simulink model "TC_RT2004_pois_CX_SNr"  (R2016b)
settings: Solver=ode4  StartTime=0.0  StopTime=simtime  FixedStep=stepsize  MaxStep=stepsize  RelTol=1e-2  EnableMultiTasking=on
values from neighbouring files (symbols this model uses):
  alphaSNrtoTH = 5    [TC_model_CX_SNr_cond_changed_parfor_opt.m]
  apr = 4    [TC_model_CX_SNr_cond_changed_parfor_opt.m]
  apt = 0.3    [TC_model_CX_SNr_cond_changed_parfor_opt.m]
  betaSNrtoTH = 0.18    [TC_model_CX_SNr_cond_changed_parfor_opt.m]
  ek = -90    [TC_model_CX_SNr_cond_changed_parfor_opt.m]
  eleak = -70    [TC_model_CX_SNr_cond_changed_parfor_opt.m]
  ena = 50    [TC_model_CX_SNr_cond_changed_parfor_opt.m]
  gkbar = 5    [TC_model_CX_SNr_cond_changed_parfor_opt.m]
  glbar = 0.05    [TC_model_CX_SNr_cond_changed_parfor_opt.m]
  gnabar = 3    [TC_model_CX_SNr_cond_changed_parfor_opt.m]
  gsynSNrtoTH = g_snr    [TC_model_CX_SNr_cond_changed_parfor_opt.m]
  gtbar = 5    [TC_model_CX_SNr_cond_changed_parfor_opt.m]
  ht0 = 0    [TC_model_CX_SNr_cond_changed_parfor_opt.m]
  htt0 = 0    [TC_model_CX_SNr_cond_changed_parfor_opt.m]
  qht = 5.5    [TC_model_CX_SNr_cond_changed_parfor_opt.m]
  s0SNrtoTH = 0    [TC_model_CX_SNr_cond_changed_parfor_opt.m]
  tadj = 1    [TC_model_CX_SNr_cond_changed_parfor_opt.m]
  vsynSNrtoTH = -85    [TC_model_CX_SNr_cond_changed_parfor_opt.m]
  vt0 = 0    [TC_model_CX_SNr_cond_changed_parfor_opt.m]
undefined symbols (not defined in the file or in its folder): jit_spk_times
settings Model: Creator=mohaghegh  LastModifiedBy=Mohammad
settings SolverCC: ZeroCrossAlgorithm=Adaptive
settings DataIOCC: LimitDataPoints=on  SaveFormat=Array
settings OptimizationCC: LifeSpan=inf
settings DebuggingCC: SolverPrmCheckMsg=warning  SFUnexpectedBacktrackingDiag=warning  SFNoUnconditionalDefaultTransitionDiag=warning  SFExecutionAtInitializationDiag=none
settings HardwareCC: ProdBitPerPointer=32  ProdBitPerSizeT=32  ProdBitPerPtrDiffT=32  ProdLargestAtomicFloat=None  ProdIntDivRoundTo=Undefined  ProdEndianess=Unspecified  ProdWordSize=32  ProdHWDeviceType=32-bit Generic
settings ModelReferenceCC: PropagateSignalLabelsOutOfModel=off
settings GRTTargetCC: TargetLangStandard=C89/C90 (ANSI)  GeneratePreprocessorConditionals=Disable all
settings ConfigComp: CovMetricSettings=dw  CovHtmlReporting=on  CovSaveCumulativeToWorkspaceVar=on  CovSaveSingleToWorkspaceVar=on  CovExternalEMLEnable=off  CovSFcnEnable=off

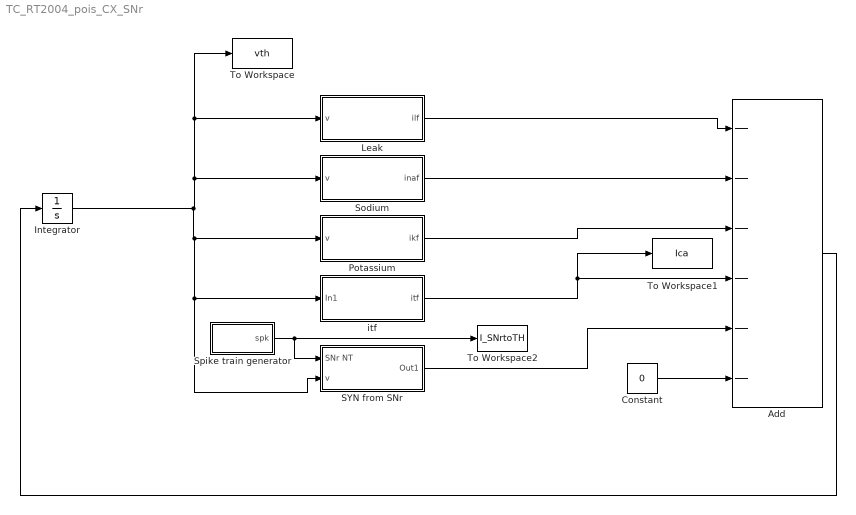
== system TC_RT2004_pois_CX_SNr ==
  Add : Sum  Inputs=------
  Constant : Constant  Value=0
  Integrator : Integrator  InitialCondition=vt0
  Leak : Subsystem
  Potassium : Subsystem
  SYN from SNr : Subsystem
  Sodium : Subsystem
  Spike train generator : Subsystem
  To Workspace : ToWorkspace  VariableName=vth  SaveFormat=Structure With Time  SampleTime=-1
  To Workspace1 : ToWorkspace  VariableName=Ica  SaveFormat=Structure With Time  SampleTime=-1
  To Workspace2 : ToWorkspace  VariableName=I_SNrtoTH  SaveFormat=Structure With Time  SampleTime=-1
  itf : Subsystem
  wires:
  Add/1 -> Integrator/1
  Leak/1(ilf) -> Add/1
  Sodium/1(inaf) -> Add/2
  Potassium/1(ikf) -> Add/3
  Integrator/1 -> SYN from SNr/2(v), itf/1(In1), Potassium/1(v), Sodium/1(v), To Workspace/1, Leak/1(v)
  SYN from SNr/1(Out1) -> Add/5
  Spike train generator/1(spk) -> To Workspace2/1, SYN from SNr/1(SNr NT)
  itf/1(itf) -> To Workspace1/1, Add/4
  Constant/1 -> Add/6

== system TC_RT2004_pois_CX_SNr/Leak ==
  v : Inport
  Constant : Constant  Value=eleak
  Gain : Gain  Gain=glbar
  Subtract : Sum  Inputs=+-
  ilf : Outport
  wires:
  v/1 -> Subtract/1
  Constant/1 -> Subtract/2
  Subtract/1 -> Gain/1
  Gain/1 -> ilf/1

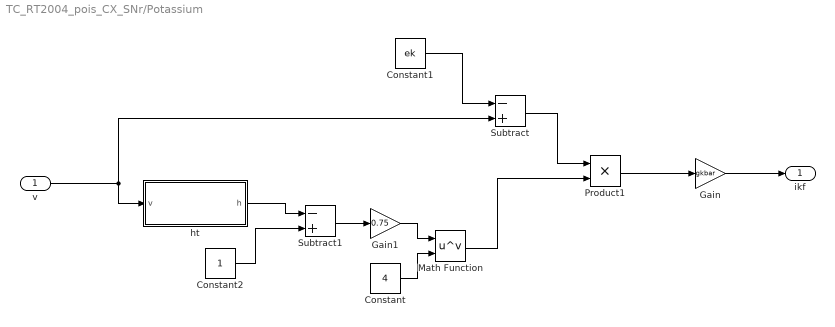
== system TC_RT2004_pois_CX_SNr/Potassium ==
  v : Inport
  Constant : Constant  Value=4
  Constant1 : Constant  Value=ek
  Constant2 : Constant
  Gain : Gain  Gain=gkbar
  Gain1 : Gain  Gain=0.75
  Math Function : Math  Operator=pow  SaturateOnIntegerOverflow=on
  Product1 : Product
  Subtract : Sum  Inputs=-+
  Subtract1 : Sum  Inputs=-+
  ht : Subsystem
  ikf : Outport
  wires:
  Gain/1 -> ikf/1
  Product1/1 -> Gain/1
  Subtract/1 -> Product1/1
  Constant1/1 -> Subtract/1
  Constant/1 -> Math Function/2
  v/1 -> ht/1(v), Subtract/2
  Math Function/1 -> Product1/2
  ht/1(h) -> Subtract1/1
  Constant2/1 -> Subtract1/2
  Subtract1/1 -> Gain1/1
  Gain1/1 -> Math Function/1

== system TC_RT2004_pois_CX_SNr/SYN from SNr ==
  SNr NT : Inport
  v : Inport  Port=2
  Add1 : Sum  Inputs=-+
  Constant : Constant  Value=vsynSNrtoTH
  Gain : Gain  Gain=gsynSNrtoTH
  Product : Product
  SNr to TH : Subsystem
  Out1 : Outport
  wires:
  Constant/1 -> Add1/1
  v/1 -> Add1/2
  Add1/1 -> Product/1
  Product/1 -> Gain/1
  Gain/1 -> Out1/1
  SNr NT/1 -> SNr to TH/1(s SNr)
  SNr to TH/1(SNr to TH cond) -> Product/2

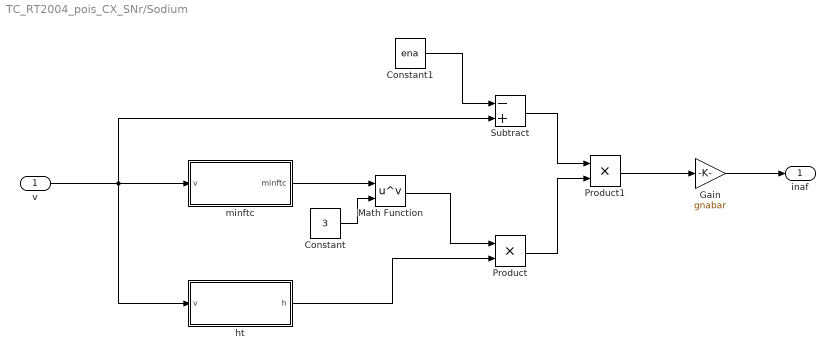
== system TC_RT2004_pois_CX_SNr/Sodium ==
  v : Inport
  Constant : Constant  Value=3
  Constant1 : Constant  Value=ena
  Gain : Gain  Gain=gnabar
  Math Function : Math  Operator=pow  SaturateOnIntegerOverflow=on
  Product : Product
  Product1 : Product
  Subtract : Sum  Inputs=-+
  ht : Subsystem
  minftc : Subsystem
  inaf : Outport
  wires:
  v/1 -> ht/1(v), minftc/1(v), Subtract/2
  minftc/1(minftc) -> Math Function/1
  Constant/1 -> Math Function/2
  Math Function/1 -> Product/1
  ht/1(h) -> Product/2
  Constant1/1 -> Subtract/1
  Subtract/1 -> Product1/1
  Product/1 -> Product1/2
  Product1/1 -> Gain/1
  Gain/1 -> inaf/1

== system TC_RT2004_pois_CX_SNr/Spike train generator ==
  Clock : Clock
  Constant : Constant  Value=jit_spk_times
  MATLAB Function : MATLAB Function  TreatAsAtomicUnit=on
  Memory : Memory
  spk : Outport
  wires:
  Clock/1 -> Memory/1, MATLAB Function/1(t1)
  Memory/1 -> MATLAB Function/2(t2)
  Constant/1 -> MATLAB Function/3(spks)
  MATLAB Function/1(y) -> spk/1

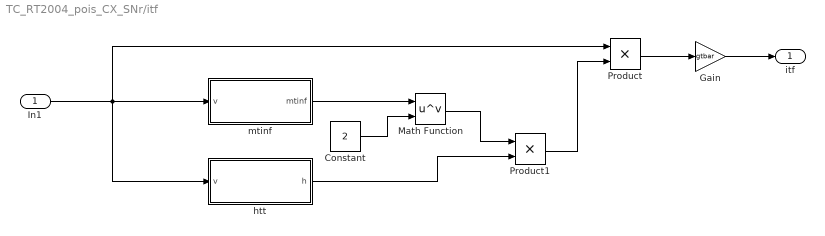
== system TC_RT2004_pois_CX_SNr/itf ==
  In1 : Inport
  Constant : Constant  Value=2
  Gain : Gain  Gain=gtbar
  Math Function : Math  Operator=pow  SaturateOnIntegerOverflow=on
  Product : Product
  Product1 : Product
  htt : Subsystem
  mtinf : Subsystem
  itf : Outport
  wires:
  In1/1 -> Product/1, mtinf/1(v), htt/1(v)
  mtinf/1(mtinf) -> Math Function/1
  Constant/1 -> Math Function/2
  Math Function/1 -> Product1/1
  htt/1(h) -> Product1/2
  Product1/1 -> Product/2
  Product/1 -> Gain/1
  Gain/1 -> itf/1

== system TC_RT2004_pois_CX_SNr/Potassium/ht ==
  v : Inport
  Divide : Product  Inputs=*/
  Gain : Gain  Gain=tadj
  Integrator : Integrator  InitialCondition=ht0
  Subtract : Sum  Inputs=-+
  hinftc : Subsystem
  tauhtc : Subsystem
  h : Outport
  wires:
  Gain/1 -> Integrator/1
  Divide/1 -> Gain/1
  tauhtc/1(tauhtc) -> Divide/2
  Subtract/1 -> Divide/1
  hinftc/1(hinftc) -> Subtract/2
  Integrator/1 -> h/1, Subtract/1
  v/1 -> tauhtc/1(v), hinftc/1(v)

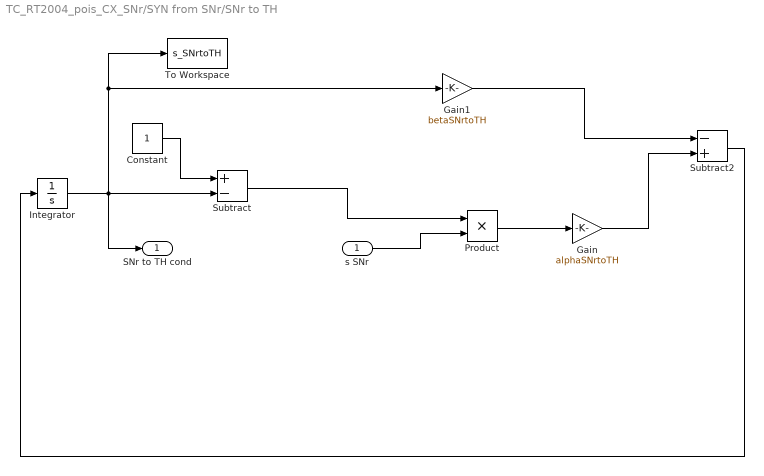
== system TC_RT2004_pois_CX_SNr/SYN from SNr/SNr to TH ==
  s SNr : Inport
  Constant : Constant
  Gain : Gain  Gain=alphaSNrtoTH
  Gain1 : Gain  Gain=betaSNrtoTH
  Integrator : Integrator  InitialCondition=s0SNrtoTH
  Product : Product
  Subtract : Sum  Inputs=+-
  Subtract2 : Sum  Inputs=-+
  To Workspace : ToWorkspace  VariableName=s_SNrtoTH  SaveFormat=Structure With Time  SampleTime=-1
  SNr to TH cond : Outport
  wires:
  Constant/1 -> Subtract/1
  Integrator/1 -> SNr to TH cond/1, To Workspace/1, Gain1/1, Subtract/2
  Subtract/1 -> Product/1
  Product/1 -> Gain/1
  Gain1/1 -> Subtract2/1
  Gain/1 -> Subtract2/2
  Subtract2/1 -> Integrator/1
  s SNr/1 -> Product/2

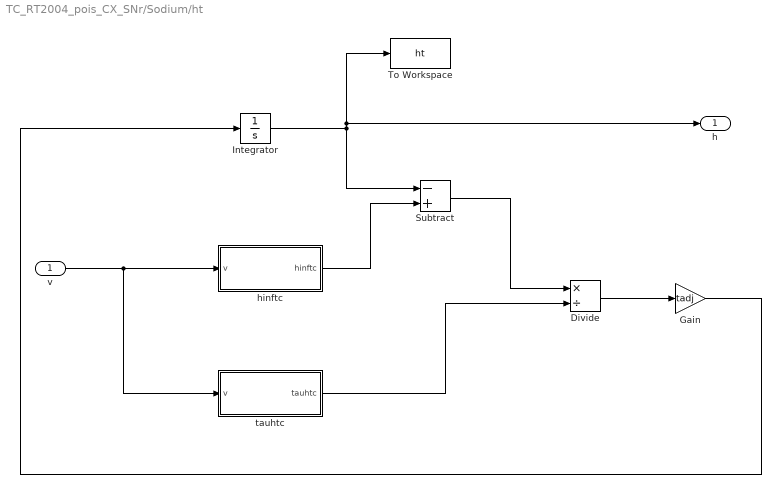
== system TC_RT2004_pois_CX_SNr/Sodium/ht ==
  v : Inport
  Divide : Product  Inputs=*/
  Gain : Gain  Gain=tadj
  Integrator : Integrator  InitialCondition=ht0
  Subtract : Sum  Inputs=-+
  To Workspace : ToWorkspace  VariableName=ht  SaveFormat=Structure With Time  SampleTime=-1
  hinftc : Subsystem
  tauhtc : Subsystem
  h : Outport
  wires:
  Gain/1 -> Integrator/1
  Divide/1 -> Gain/1
  tauhtc/1(tauhtc) -> Divide/2
  Subtract/1 -> Divide/1
  hinftc/1(hinftc) -> Subtract/2
  Integrator/1 -> To Workspace/1, h/1, Subtract/1
  v/1 -> tauhtc/1(v), hinftc/1(v)

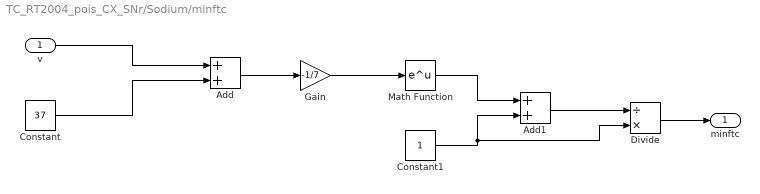
== system TC_RT2004_pois_CX_SNr/Sodium/minftc ==
  v : Inport
  Add : Sum
  Add1 : Sum
  Constant : Constant  Value=37
  Constant1 : Constant
  Divide : Product  Inputs=/*
  Gain : Gain  Gain=-1/7
  Math Function : Math  SaturateOnIntegerOverflow=on
  minftc : Outport
  wires:
  v/1 -> Add/1
  Constant/1 -> Add/2
  Add/1 -> Gain/1
  Gain/1 -> Math Function/1
  Math Function/1 -> Add1/1
  Add1/1 -> Divide/1
  Constant1/1 -> Divide/2, Add1/2
  Divide/1 -> minftc/1

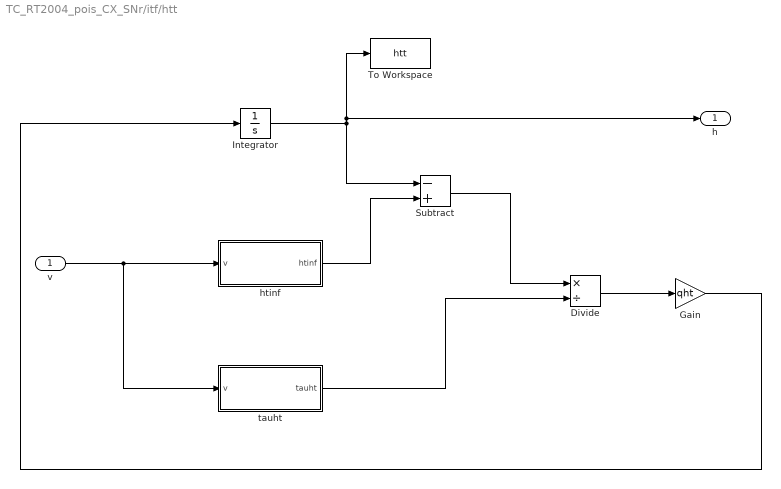
== system TC_RT2004_pois_CX_SNr/itf/htt ==
  v : Inport
  Divide : Product  Inputs=*/
  Gain : Gain  Gain=qht
  Integrator : Integrator  InitialCondition=htt0
  Subtract : Sum  Inputs=-+
  To Workspace : ToWorkspace  VariableName=htt  SaveFormat=Structure With Time  SampleTime=-1
  htinf : Subsystem
  tauht : Subsystem
  h : Outport
  wires:
  v/1 -> tauht/1(v), htinf/1(v)
  Integrator/1 -> To Workspace/1, h/1, Subtract/1
  htinf/1(htinf) -> Subtract/2
  Subtract/1 -> Divide/1
  tauht/1(tauht) -> Divide/2
  Divide/1 -> Gain/1
  Gain/1 -> Integrator/1

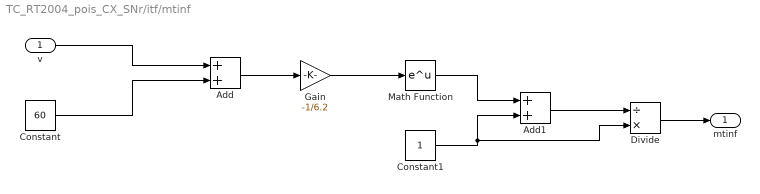
== system TC_RT2004_pois_CX_SNr/itf/mtinf ==
  v : Inport
  Add : Sum
  Add1 : Sum
  Constant : Constant  Value=60
  Constant1 : Constant
  Divide : Product  Inputs=/*
  Gain : Gain  Gain=-1/6.2
  Math Function : Math  SaturateOnIntegerOverflow=on
  mtinf : Outport
  wires:
  Divide/1 -> mtinf/1
  Constant1/1 -> Add1/2, Divide/2
  Add1/1 -> Divide/1
  Math Function/1 -> Add1/1
  Gain/1 -> Math Function/1
  Add/1 -> Gain/1
  Constant/1 -> Add/2
  v/1 -> Add/1

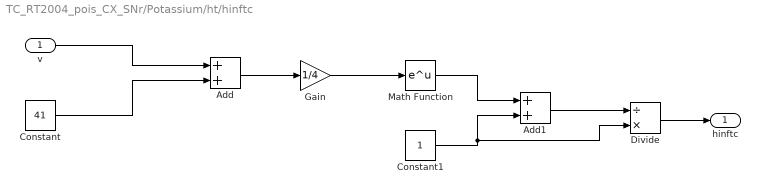
== system TC_RT2004_pois_CX_SNr/Potassium/ht/hinftc ==
  v : Inport
  Add : Sum
  Add1 : Sum
  Constant : Constant  Value=41
  Constant1 : Constant
  Divide : Product  Inputs=/*
  Gain : Gain  Gain=1/4
  Math Function : Math  SaturateOnIntegerOverflow=on
  hinftc : Outport
  wires:
  v/1 -> Add/1
  Constant/1 -> Add/2
  Add/1 -> Gain/1
  Gain/1 -> Math Function/1
  Math Function/1 -> Add1/1
  Add1/1 -> Divide/1
  Constant1/1 -> Divide/2, Add1/2
  Divide/1 -> hinftc/1

== system TC_RT2004_pois_CX_SNr/Potassium/ht/tauhtc ==
  v : Inport
  Add : Sum
  Constant : Constant
  Divide : Product  Inputs=*/
  ah : Subsystem
  bh : Subsystem
  tauhtc : Outport
  wires:
  v/1 -> bh/1(v), ah/1(v)
  ah/1(ah) -> Add/1
  bh/1(bh) -> Add/2
  Constant/1 -> Divide/1
  Add/1 -> Divide/2
  Divide/1 -> tauhtc/1

== system TC_RT2004_pois_CX_SNr/Sodium/ht/hinftc ==
  v : Inport
  Add : Sum
  Add1 : Sum
  Constant : Constant  Value=41
  Constant1 : Constant
  Divide : Product  Inputs=/*
  Gain : Gain  Gain=1/4
  Math Function : Math  SaturateOnIntegerOverflow=on
  hinftc : Outport
  wires:
  v/1 -> Add/1
  Constant/1 -> Add/2
  Add/1 -> Gain/1
  Gain/1 -> Math Function/1
  Math Function/1 -> Add1/1
  Add1/1 -> Divide/1
  Constant1/1 -> Divide/2, Add1/2
  Divide/1 -> hinftc/1

== system TC_RT2004_pois_CX_SNr/Sodium/ht/tauhtc ==
  v : Inport
  Add : Sum
  Constant : Constant
  Divide : Product  Inputs=*/
  ah : Subsystem
  bh : Subsystem
  tauhtc : Outport
  wires:
  v/1 -> bh/1(v), ah/1(v)
  ah/1(ah) -> Add/1
  bh/1(bh) -> Add/2
  Constant/1 -> Divide/1
  Add/1 -> Divide/2
  Divide/1 -> tauhtc/1

== system TC_RT2004_pois_CX_SNr/itf/htt/htinf ==
  v : Inport
  Add : Sum
  Add1 : Sum
  Constant : Constant  Value=84
  Constant1 : Constant
  Divide : Product  Inputs=/*
  Gain : Gain  Gain=1/4
  Math Function : Math  SaturateOnIntegerOverflow=on
  htinf : Outport
  wires:
  v/1 -> Add/1
  Constant/1 -> Add/2
  Add/1 -> Gain/1
  Gain/1 -> Math Function/1
  Math Function/1 -> Add1/1
  Add1/1 -> Divide/1
  Constant1/1 -> Divide/2, Add1/2
  Divide/1 -> htinf/1

== system TC_RT2004_pois_CX_SNr/itf/htt/tauht ==
  v : Inport
  Add : Sum
  Add1 : Sum
  Constant : Constant  Value=25
  Constant1 : Constant  Value=28
  Gain : Gain  Gain=-1/10.5
  Gain1 : Gain  Gain=apt
  Math Function : Math  SaturateOnIntegerOverflow=on
  tauht : Outport
  wires:
  v/1 -> Add/1
  Constant/1 -> Add/2
  Add/1 -> Gain/1
  Gain/1 -> Math Function/1
  Constant1/1 -> Add1/2
  Math Function/1 -> Gain1/1
  Gain1/1 -> Add1/1
  Add1/1 -> tauht/1

== system TC_RT2004_pois_CX_SNr/Potassium/ht/tauhtc/ah ==
  v : Inport
  Add : Sum
  Constant : Constant  Value=46
  Gain : Gain  Gain=-1/18
  Gain1 : Gain  Gain=0.128
  Math Function : Math  SaturateOnIntegerOverflow=on
  ah : Outport
  wires:
  v/1 -> Add/1
  Constant/1 -> Add/2
  Add/1 -> Gain/1
  Gain/1 -> Math Function/1
  Math Function/1 -> Gain1/1
  Gain1/1 -> ah/1

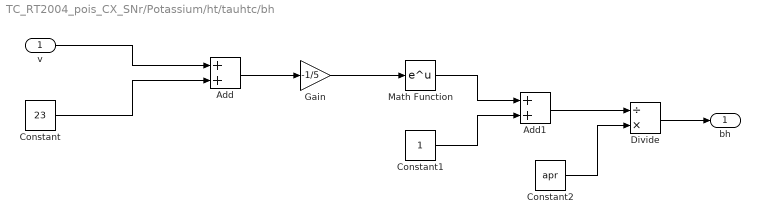
== system TC_RT2004_pois_CX_SNr/Potassium/ht/tauhtc/bh ==
  v : Inport
  Add : Sum
  Add1 : Sum
  Constant : Constant  Value=23
  Constant1 : Constant
  Constant2 : Constant  Value=apr
  Divide : Product  Inputs=/*
  Gain : Gain  Gain=-1/5
  Math Function : Math  SaturateOnIntegerOverflow=on
  bh : Outport
  wires:
  v/1 -> Add/1
  Constant/1 -> Add/2
  Add/1 -> Gain/1
  Gain/1 -> Math Function/1
  Math Function/1 -> Add1/1
  Add1/1 -> Divide/1
  Constant1/1 -> Add1/2
  Divide/1 -> bh/1
  Constant2/1 -> Divide/2

== system TC_RT2004_pois_CX_SNr/Sodium/ht/tauhtc/ah ==
  v : Inport
  Add : Sum
  Constant : Constant  Value=46
  Gain : Gain  Gain=-1/18
  Gain1 : Gain  Gain=0.128
  Math Function : Math  SaturateOnIntegerOverflow=on
  ah : Outport
  wires:
  v/1 -> Add/1
  Constant/1 -> Add/2
  Add/1 -> Gain/1
  Gain/1 -> Math Function/1
  Math Function/1 -> Gain1/1
  Gain1/1 -> ah/1

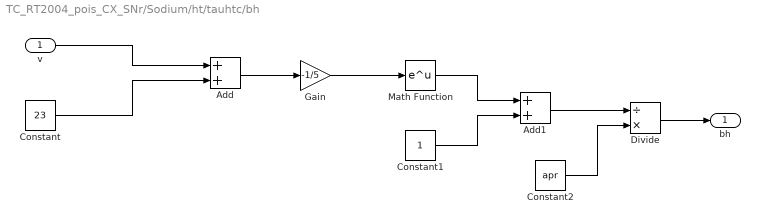
== system TC_RT2004_pois_CX_SNr/Sodium/ht/tauhtc/bh ==
  v : Inport
  Add : Sum
  Add1 : Sum
  Constant : Constant  Value=23
  Constant1 : Constant
  Constant2 : Constant  Value=apr
  Divide : Product  Inputs=/*
  Gain : Gain  Gain=-1/5
  Math Function : Math  SaturateOnIntegerOverflow=on
  bh : Outport
  wires:
  v/1 -> Add/1
  Constant/1 -> Add/2
  Add/1 -> Gain/1
  Gain/1 -> Math Function/1
  Math Function/1 -> Add1/1
  Add1/1 -> Divide/1
  Constant1/1 -> Add1/2
  Divide/1 -> bh/1
  Constant2/1 -> Divide/2

== matlab function TC_RT2004_pois_CX_SNr/Spike train generator/MATLAB Function ==
  data: t1 input; y output; t2 input; spks input
function y = fcn(t1,t2,spks)
%#codegen

y = sum(spks<t1 & spks>t2);
